simulink model "SPL"  (R2024a)
settings: Solver=VariableStepAuto  StartTime=0.0  StopTime=10  RelTol=1e-3
values from neighbouring files (symbols this model uses):
  A = [A1, A2 ... (first row only)    [SPL_1.m]
  G = [ ... (first row only)    [SPL_1.m]
settings Model: Creator=isabe  LastModifiedBy=isabe

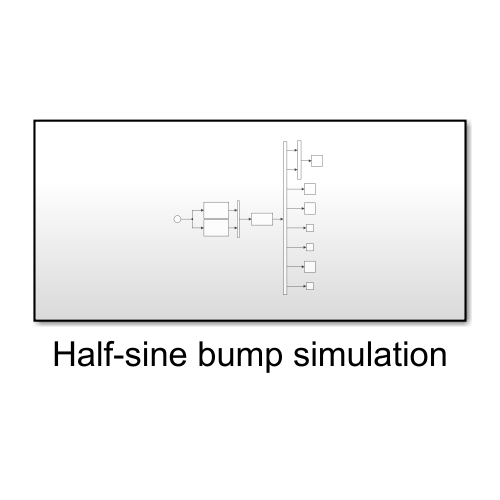
[thumbnail: Simulink's stored preview of the top-level diagram]
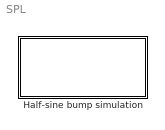
== system SPL ==
  Half-sine bump simulation : Subsystem

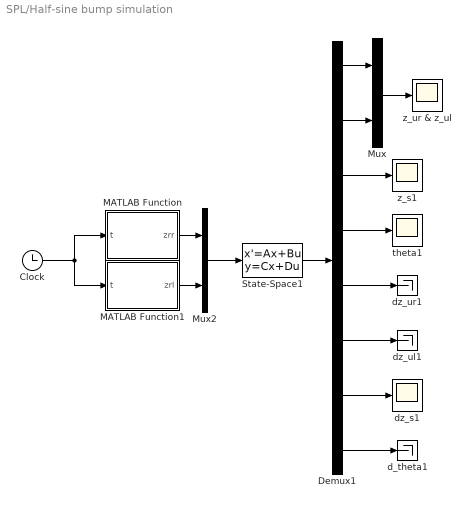
== system SPL/Half-sine bump simulation ==
  Clock : Clock
  Demux1 : Demux  Outputs=8
  MATLAB Function : MATLAB Function  TreatAsAtomicUnit=on
  MATLAB Function1 : MATLAB Function  TreatAsAtomicUnit=on
  Mux : Mux  Inputs=2
  Mux2 : Mux  Inputs=2
  State-Space1 : StateSpace  A=A  B=G  C=eye(8)  D=zeros(8,2)  InitialCondition=zeros(8,1)
  d_theta1 : Terminator
  dz_s1 : Scope
  dz_ul1 : Terminator
  dz_ur1 : Terminator
  theta1 : Scope
  z_s1 : Scope
  z_ur & z_ul : Scope
  wires:
  MATLAB Function/1(zrr) -> Mux2/1
  Clock/1 -> MATLAB Function/1(t), MATLAB Function1/1(t)
  MATLAB Function1/1(zrl) -> Mux2/2
  Demux1/7 -> dz_s1/1
  Demux1/5 -> dz_ur1/1
  Demux1/4 -> theta1/1
  Demux1/3 -> z_s1/1
  Mux2/1 -> State-Space1/1
  State-Space1/1 -> Demux1/1
  Demux1/6 -> dz_ul1/1
  Demux1/8 -> d_theta1/1
  Demux1/2 -> Mux/2
  Demux1/1 -> Mux/1
  Mux/1 -> z_ur & z_ul/1

== matlab function SPL/Half-sine bump simulation/MATLAB Function1 ==
  data: t input; zrl output
function zrl  =  MATLAB_Function(t)
    a_r=0.05; a_l=0.08; b=0.5; V=10;
    t1_r=1.0; t1_l=1.3;
    T = b/V; omega = 2*pi*V/b;
    
    if t >= t1_l && t <= t1_l + T
        zrl = (a_l/2)*(1 - cos(omega*(t - t1_l)));
    else
        zrl = 0;
    end
end

== matlab function SPL/Half-sine bump simulation/MATLAB Function ==
  data: t input; zrr output
function zrr  =  MATLAB_Function(t)
    a_r=0.05; a_l=0.08; b=0.5; V=10;
    t1_r=1.0; t1_l=1.3;
    T = b/V; omega = 2*pi*V/b;
    
    if t >= t1_r && t <= t1_r + T
        zrr = (a_r/2)*(1 - cos(omega*(t - t1_r)));
    else
        zrr = 0;
    end
end
